simulink library "NCS_Library"  (R2019a)
settings: Solver=VariableStepAuto  StartTime=0.0  StopTime=10.0  RelTol=1e-3
values from neighbouring files (symbols this model uses):
  A = 10    [Parameter.m]
  band = 100000000    [Parameter.m]
  BER = 0    [Parameter.m]
  c = 5000000    [Parameter.m]
  c1 = 4.33    [Parameter.m]
  c2 = 3.16    [Parameter.m]
  CAN2EthernetDelay = 0.000    (= 0)    [Parameter.m]
  cR = 1.5*10^-3    (= 0.0015)    [Parameter.m]
  cw = (cwE * 2 + cwM * (nW_ges-2))/nW_ges    (= 0.1475)    [Parameter.m]
  cwE = 0.35    [Parameter.m]
  cwM = 0.08    [Parameter.m]
  Cycle_Controller = 0    [Parameter.m]
  CyclePLC = 24/1000    (= 0.024)    [Parameter.m]
  d = 800000    [Parameter.m]
  Dr = 0.92    [Parameter.m]
  Ethernet2CANDelay = 0.005    [Parameter.m]
  F_konst = 70892    [Parameter.m]
  FA = 100000    [Parameter.m]
  FB_WB_max = 10000    [Parameter.m]
  FBel_an = iG*nG*F_KZmax*nBan*R_mR/(Dr/2)    (= 28197.4297239)    [Parameter.m]
  FBel_frei = iG*nG*F_KZmax*nBfrei*R_mW/(Dr/2)    (= 29270.6882948)    [Parameter.m]
  Fmaxdyn = 300000    [Parameter.m]
  g = 9.81    [Parameter.m]
  i = 0    [Parameter.m]
  J = 1/2*mA*(Dr/2)^2    (= 158.7)    [Parameter.m]
  k1 = 0.095    [Parameter.m]
  k2 = 9.26/3.6    (= 2.57222222222)    [Parameter.m]
  k3 = 4.63/3.6    (= 1.28611111111)    [Parameter.m]
  mges = 58000    [Parameter.m]
  mu = [mu1 mu2]    [Parameter.m]
  muBel1 = 0.42    [Parameter.m]
  muBel2 = 0.36    [Parameter.m]
  n = 0.001    [Parameter.m]
  n_Mg = 4    [Parameter.m]
  n_WB = 4    [Parameter.m]
  nA = 4    [Parameter.m]
  nBan = 2    [Parameter.m]
  nBfrei = 3    [Parameter.m]
  nM = 4    [Parameter.m]
  nW_an = 4    [Parameter.m]
  P_max = 8200000    [Parameter.m]
  Q = 10    [Parameter.m]
  r_reib = 600    [Parameter.m]
  rho = 1.08    [Parameter.m]
  rhoL = 1.225    [Parameter.m]
  Size = 8    [Parameter.m]
  slip = [s1 s2]    [Parameter.m]
  tol = 0.05    [Parameter.m]
  v00 = 100/3.6    (= 27.7777777778)    [Parameter.m]
  v_grenz = 60/3.6    (= 16.6666666667)    [Parameter.m]
  v_opt = 75/3.6    (= 20.8333333333)    [Parameter.m]
  W_opt = 0.5    [Parameter.m]
  WB = 1    [Parameter.m]
  y_opt = sqrt(W_opt)/((1+sqrt(W_opt))^2+W_opt)    [Parameter.m]
undefined symbols (not defined in the file or in its folder): BUSCapacity, CableLength, controlGate, D_dyn, D_mg, EnableBurst, EnableToF, entity, Entity_out, Gate, Gate_4, Gate_5, Gate_ACK, Gate_copy, Gate_RX, getData, gettime, I_dyn, I_mg, m, magnitude, P_dyn, P_mg, ReadAttributes, readdata, ReadData, ReadSize, sigbuilder_block, Timeout, ToB, ToF, v0, v_d, v_soll
libraries: simulink x176, $bdroot x102
(part 8 of 12)

== system NCS_Library/Network/CAN/Logik/Slow_to_Fast/Logic Takt ==
  In : Inport
  Entity Takt : EntityGenerator  OutputPortMessageModes=m  TimeSource=Signal port  Period=7  AttributeName=entity  EntityTypeName=gate  EntityPriority=10  DataInitialValue=1
      settings: InputPortMap=u1
  Entity Terminator13 : EntityTerminator  InputPortMessageModes=m
  Gate : EntityGate  InputPortMessageModes=m,m  OutputPortMessageModes=m
  Offset [s] : Constant  Value=Offset
  Server : EntityServer  InputPortMessageModes=m  OutputPortMessageModes=m  Capacity=1  ServiceTimeValue=0  EntryAction=Gate(0);
  Server Offset : EntityServer  InputPortMessageModes=n,m  OutputPortMessageModes=m  Capacity=inf  ServiceTimeSource=Signal port  ServiceTimeValue=5
      settings: InputPortMap=u0,u2
  Server Takt : EntityServer  InputPortMessageModes=m  OutputPortMessageModes=m  Capacity=1  ServiceTimeValue=0.001  ServiceTimeAttributeName=CommDelay  EntryAction=Gate(Copy_on);  ExitAction=Gate(0);  SortingAttributeName=ID
  Simulink Function3 : Subsystem  TreatAsAtomicUnit=on
  Takt_fast [s] : Constant  Value=Takt_fast
  Out : Outport
  wires:
  Server/1 -> Out/1
  Gate/1 -> Server/1
  In/1 -> Gate/2
  Simulink Function3/1(ctrl) -> Gate/1
  Entity Takt/1 -> Server Offset/2
  Server Offset/1 -> Server Takt/1
  Server Takt/1 -> Entity Terminator13/1
  Takt_fast [s]/1 -> Entity Takt/1
  Offset [s]/1 -> Server Offset/1

== system NCS_Library/Network/CAN/Logik/Slow_to_Fast/Measurement ==
  measure : Inport
  Buffer_Measure : EntityQueue  InputPortMessageModes=m  OutputPortMessageModes=n,m  Capacity=1000  QueueType=LIFO  NumberEntitiesInBlock=on
      settings: OutputPortMap=o1,o5
  Detect Change : simulink/Logic and Bit Operations/Detect Change  vinit=0  OutDataTypeStr=boolean
  Digital Clock2 : DigitalClock  SampleTime=0.01
  Enabled Subsystem : Subsystem  TreatAsAtomicUnit=on
  Entity Replicator5 : EntityReplicator  InputPortMessageModes=m  OutputPortMessageModes=m,m
  Entity Terminator8 : EntityTerminator  InputPortMessageModes=m  EntryAction=getData(entity.Time)  NumberEntitiesArrived=on
      settings: OutputPortMap=o0
  Fast Takt : Subsystem
  Scope{,1,3,6} (4 alike) : Scope
  Simulink Function6 : Subsystem  TreatAsAtomicUnit=on
  Out : Outport
  wires:
  Digital Clock2/1 -> Enabled Subsystem/1(time_arrived)
  Simulink Function6/1(time) -> Enabled Subsystem/2(time), Scope3/1
  Detect Change/1 -> Enabled Subsystem/Enable
  Buffer_Measure/2 -> Fast Takt/1(In)
  Fast Takt/1(Out) -> Entity Replicator5/1
  Entity Terminator8/1 -> Detect Change/1, Scope6/1
  measure/1 -> Buffer_Measure/1
  Buffer_Measure/1 -> Scope1/1
  Enabled Subsystem/1(delay) -> Scope/1
  Entity Replicator5/2 -> Entity Terminator8/1
  Entity Replicator5/1 -> Out/1

== system NCS_Library/Network/CAN/Logik/Slow_to_Fast/Simulink Function1 ==
  Entity_out : TriggerPort  TriggerType=function-call  IsSimulinkFunction=on  FunctionName=Entity_out  FunctionVisibility=scoped  VariantControl=Variant
  Message Send : MessageSend  OutputPortMessageModes=m
      settings: InputPortMap=u1
  u : ArgIn  DisableCoverage=on  ArgumentName=u
  ctrl : Outport
  wires:
  u/1 -> Message Send/1
  Message Send/1 -> ctrl/1

== system NCS_Library/Network/CAN/Logik/Slow_to_Fast/Simulink Function3 ==
  Entity_in : TriggerPort  TriggerType=function-call  IsSimulinkFunction=on  FunctionName=Entity_in  FunctionVisibility=scoped  VariantControl=Variant
  Message Send : MessageSend  OutputPortMessageModes=m
      settings: InputPortMap=u1
  u : ArgIn  DisableCoverage=on  ArgumentName=u
  ctrl : Outport
  wires:
  Message Send/1 -> ctrl/1
  u/1 -> Message Send/1

== system NCS_Library/Network/ETB/Burst Device/Protocl Stack/TRDP PD ==
  note: Transmit
  note: Receive
  InFromSDTv2 : Inport
  Paramter : Inport  Port=2
  InFromUDP : Inport  Port=3
  Bus Selector : BusSelector  OutputSignals=T_Tx,SDTv2,msgType,Destination
  Bus Selector1 : BusSelector  OutputSignals=Address,Port,ReplyAddress
  Compare To Zero : simulink/Logic and Bit Operations/Compare To Zero  relop=>  OutDataTypeStr=boolean
  Constant : Constant  Value=0.0
  Constant2 : Constant
  Data Type Conversion : DataTypeConversion  OutDataTypeStr=uint8
  Detect Change : simulink/Logic and Bit Operations/Detect Change  vinit=0  OutDataTypeStr=boolean
  Display4 : Display
  Enabled Subsystem1 : Subsystem  TreatAsAtomicUnit=on
  Entity Server : EntityServer  InputPortMessageModes=n,m  OutputPortMessageModes=n,m  Capacity=1  ServiceTimeSource=Signal port  EntryAction=ReadData( entity.msgType, entity.ReplyAddress, entity.Source);  NumberEntitiesDeparted=on
      settings: InputPortMap=u0,u2  OutputPortMap=o0,o9
  Entity Server1 : EntityServer  InputPortMessageModes=m  OutputPortMessageModes=n,m  Capacity=1  ServiceTimeValue=0  EntryAction=[entity.SEQ, entity.msgType, entity.Destination, entity.Source, entity.CheckBit, entity.Data, entity.Port, entity.ReplyAddress] = SetAttributes(entity.SSC, entity.Data);  NumberEntitiesDeparted=on
      settings: OutputPortMap=o0,o9
  Message Send : MessageSend  OutputPortMessageModes=m  ShowEnablePort=on
      settings: InputPortMap=e0,u1
  Simulink Function : Subsystem  TreatAsAtomicUnit=on
  Simulink Function1 : Subsystem  TreatAsAtomicUnit=on
  Terminator{,1..3} (4 alike) : Terminator
  OutToSDTv2 : Outport
  TRM : Outport  Port=2
  #Transmit : Outport  Port=3
  msgType_transmit : Outport  Port=4
  #Receive : Outport  Port=5
  msgType_receive : Outport  Port=6
  OutToUDP : Outport  Port=7
  wires:
  Constant2/1 -> Message Send/2
  Message Send/1 -> TRM/1
  Bus Selector1/3 -> Simulink Function/5(ReplyAddress)  "<ReplyAddress>"
  Bus Selector1/2 -> Simulink Function/4(UDP)  "<Port>"
  Bus Selector1/1 -> Simulink Function/3(Source)  "<Address>"
  Bus Selector/3 -> Data Type Conversion/1  "<msgType>"
  Entity Server1/1 -> #Transmit/1
  Entity Server/1 -> Detect Change/1, #Receive/1
  Detect Change/1 -> Enabled Subsystem1/Enable
  Simulink Function1/2(ReplyAddress) -> Enabled Subsystem1/2(ReplyAddress)
  Simulink Function1/1(msgType) -> Enabled Subsystem1/1(msgType), msgType_receive/1
  InFromSDTv2/1 -> Entity Server1/1
  Entity Server1/2 -> OutToUDP/1
  Paramter/1 -> Bus Selector/1, Bus Selector1/1
  Constant/1 -> Entity Server/1
  Entity Server/2 -> OutToSDTv2/1
  Compare To Zero/1 -> Display4/1, Message Send/1
  Bus Selector/4 -> Simulink Function/2(Destination)  "<Destination>"
  InFromUDP/1 -> Entity Server/2
  Enabled Subsystem1/1(msgTypeReply) -> Terminator/1
  Enabled Subsystem1/2(DestinationReply) -> Terminator1/1
  Bus Selector/1 -> Terminator2/1  "<T_Tx>"
  Bus Selector/2 -> Terminator3/1  "<SDTv2>"
  Data Type Conversion/1 -> Compare To Zero/1, msgType_transmit/1, Simulink Function/1(msgType)

== system NCS_Library/Network/ETB/Controller Interface/Subsystem/Transport Layers ==
  InFromApplication4 : Inport
  InFromApplication3 : Inport  Port=2
  InFromApplication2 : Inport  Port=3
  InFromApplication1 : Inport  Port=4
  Parameter : Inport  Port=5
  RxFromBus : Inport  Port=6
  CycleRx : EntityServer  InputPortMessageModes=m  OutputPortMessageModes=m  Capacity=100  ServiceTimeValue=CycleRx
  CycleTx : EntityServer  InputPortMessageModes=m  OutputPortMessageModes=m  Capacity=100  ServiceTimeValue=CycleTx
  Entity Generator1 : EntityGenerator  InputPortMessageModes=m  OutputPortMessageModes=m  GenerationMethod=Event-based  TimeSource=Signal port  GenerateEntityAtSimulationStart=off  EntityType=Bus object  EntityTypeName=Ethernet_Entity
      settings: InputPortMap=u0
  Entity Replicator : EntityReplicator  InputPortMessageModes=m  OutputPortMessageModes=m,m,m,m  NumberReplicas=3
      settings: OutputPortMap=o0,o1,o2,o3
  Entity Terminator{3..6} (4 alike) : EntityTerminator  InputPortMessageModes=m
  Ground1 : Ground
  IP : $bdroot/Network/ETB/OSI Layers/IP  SystemSampleTime=-1
  MAC Controller : $bdroot/Network/ETB/OSI Layers/MAC Controller  SystemSampleTime=-1
  Parameter1 : InportShadow  Port=5
  Terminator : Terminator
  Terminator1 : Terminator
  UDP Multi-Port : $bdroot/Network/ETB/OSI Layers/UDP Multi-Port  SystemSampleTime=-1
  OutToApplication4 : Outport
  OutToApplication3 : Outport  Port=2
  OutToApplication2 : Outport  Port=3
  OutToApplication1 : Outport  Port=4
  Delay : Outport  Port=5
  #damaged : Outport  Port=6
  TxToBus : Outport  Port=7
  wires:
  Parameter/1 -> MAC Controller/2
  RxFromBus/1 -> MAC Controller/3
  MAC Controller/4 -> TxToBus/1
  Parameter1/1 -> IP/2
  MAC Controller/2 -> Terminator/1  "#collision"
  MAC Controller/3 -> Terminator1/1  "Retry"
  UDP Multi-Port/9 -> IP/1
  IP/1 -> UDP Multi-Port/9
  UDP Multi-Port/1 -> OutToApplication1/1
  Entity Generator1/1 -> Entity Replicator/1
  UDP Multi-Port/5 -> Entity Terminator3/1
  UDP Multi-Port/6 -> Entity Terminator4/1
  UDP Multi-Port/7 -> Entity Terminator5/1
  UDP Multi-Port/8 -> Entity Terminator6/1
  Ground1/1 -> Entity Generator1/1
  InFromApplication1/1 -> UDP Multi-Port/1
  InFromApplication2/1 -> UDP Multi-Port/2
  InFromApplication3/1 -> UDP Multi-Port/3
  InFromApplication4/1 -> UDP Multi-Port/4
  Entity Replicator/1 -> UDP Multi-Port/5
  Entity Replicator/2 -> UDP Multi-Port/6
  Entity Replicator/3 -> UDP Multi-Port/7
  Entity Replicator/4 -> UDP Multi-Port/8
  UDP Multi-Port/3 -> OutToApplication3/1
  UDP Multi-Port/4 -> OutToApplication4/1
  UDP Multi-Port/2 -> OutToApplication2/1
  IP/4 -> CycleTx/1
  CycleTx/1 -> MAC Controller/1
  CycleRx/1 -> IP/3
  MAC Controller/1 -> CycleRx/1
  IP/3 -> Delay/1  "delay"
  IP/2 -> #damaged/1

== system NCS_Library/Network/ETB/ED/Protocol Stack/Simulink Function ==
  f : TriggerPort  TriggerType=function-call  IsSimulinkFunction=on  FunctionName=ReadSize  FunctionVisibility=scoped  VariantControl=(inherit)
  u : ArgIn  DisableCoverage=on  ArgumentName=Size
  Out1 : Outport
  wires:
  u/1 -> Out1/1

== system NCS_Library/Network/ETB/ED/Protocol Stack/Subsystem ==
  Signal : Inport
  Data : Inport  Port=2
  In3 : Inport  Port=3
  Phase : Inport  Port=4
  In5 : Inport  Port=5
  In6 : Inport  Port=6
  In7 : Inport  Port=7
  In8 : Inport  Port=8
  In9 : Inport  Port=9
  delay : Inport  Port=10
  #collision : Inport  Port=11
  Retry : Inport  Port=12
  SDTv2 : Inport  Port=13
  Bus Creator1 : BusCreator  Commented=on  Inputs=13
  Data Type Conversion{,1..6} (7 alike) : DataTypeConversion  OutDataTypeStr=double
  Detect Change : simulink/Logic and Bit Operations/Detect Change  vinit=0  OutDataTypeStr=boolean
  Out1 : Outport
  wires:
  SDTv2/1 -> Bus Creator1/13  "SDTv2"
  Data Type Conversion/1 -> Bus Creator1/6  "msgType_transmit"
  Signal/1 -> Bus Creator1/1
  Data Type Conversion5/1 -> Bus Creator1/9  "#damaged"
  Data Type Conversion6/1 -> Bus Creator1/7  "#Receive"
  Data Type Conversion1/1 -> Bus Creator1/5  "#Transmit"
  In7/1 -> Data Type Conversion6/1
  Data Type Conversion3/1 -> Bus Creator1/3  "SSC"
  Data Type Conversion2/1 -> Bus Creator1/8  "msgType_receive"
  Data Type Conversion4/1 -> Bus Creator1/12  "Retry"
  Detect Change/1 -> Data Type Conversion4/1
  In6/1 -> Data Type Conversion/1
  Data/1 -> Bus Creator1/2
  In9/1 -> Data Type Conversion5/1
  In3/1 -> Data Type Conversion3/1
  #collision/1 -> Bus Creator1/11
  In8/1 -> Data Type Conversion2/1
  In5/1 -> Data Type Conversion1/1
  delay/1 -> Out1/1, Bus Creator1/10
  Retry/1 -> Detect Change/1
  Phase/1 -> Bus Creator1/4

== system NCS_Library/Network/ETB/ED/User Interface/Subsystem2 ==
  In1 : Inport
  MATLAB Function : MATLAB Function  TreatAsAtomicUnit=on
  Out1 : Outport
  wires:
  MATLAB Function/1(y) -> Out1/1
  In1/1 -> MATLAB Function/1(u)

== system NCS_Library/Network/ETB/OSI Layers/Application/Edit Paramter ==
  UDP_Port : Inport
  Parameter : Inport  Port=2
  Bus Creator : BusCreator  Inputs=8
  Bus Selector : BusSelector  OutputSignals=Address,Destination,Subscribe,ReplyAddress,Port,T_Tx,msgType,SDTv2
  Display : Display
  MATLAB Function : MATLAB Function  TreatAsAtomicUnit=on
  MATLAB Function1 : MATLAB Function  TreatAsAtomicUnit=on
  MATLAB Function2 : MATLAB Function  TreatAsAtomicUnit=on
  MATLAB Function3 : MATLAB Function  TreatAsAtomicUnit=on
  Terminator : Terminator
  UDP_Port{1..4} (4 alike) : InportShadow
  Parameter_edited : Outport
  wires:
  Parameter/1 -> Bus Selector/1
  Bus Creator/1 -> Parameter_edited/1
  Bus Selector/6 -> MATLAB Function1/2(In)  "<T_Tx>"
  Bus Selector/3 -> Bus Creator/3  "<Subscribe>"
  Bus Selector/1 -> Bus Creator/1  "<Address>"
  Bus Selector/8 -> MATLAB Function3/2(In)  "<SDTv2>"
  Bus Selector/2 -> MATLAB Function/2(U)  "<Destination>"
  MATLAB Function/1(y) -> Display/1, Bus Creator/2  "Destination"
  UDP_Port/1 -> MATLAB Function/1(UDP)  "Port"
  UDP_Port1/1 -> Bus Creator/5  "Port"
  Bus Selector/5 -> Terminator/1  "<Port>"
  MATLAB Function1/1(Value) -> Bus Creator/6  "T_Tx"
  UDP_Port2/1 -> MATLAB Function1/1(Port)  "Port"
  MATLAB Function2/1(Value) -> Bus Creator/7  "msgType"
  Bus Selector/7 -> MATLAB Function2/2(In)  "<msgType>"
  UDP_Port3/1 -> MATLAB Function2/1(Port)  "Port"
  MATLAB Function3/1(Value) -> Bus Creator/8  "SDTv2"
  UDP_Port4/1 -> MATLAB Function3/1(Port)  "Port"
  Bus Selector/4 -> Bus Creator/4  "<ReplyAddress>"

== system NCS_Library/Network/ETB/OSI Layers/Application/Receive Sensor Data ==
  Parameter : Inport
  InFromUDP : Inport  Port=2
  Bus Selector : BusSelector  OutputSignals=SDTv2,T_Tx,msgType
  Entity Terminator : EntityTerminator  InputPortMessageModes=m
  Ground : Ground
  Ground2 : Ground
  SDTv2 : $bdroot/Network/ETB/OSI Layers/SDTv2  SystemSampleTime=-1
  TRDP PD : $bdroot/Network/ETB/OSI Layers/TRDP PD  SystemSampleTime=-1
  Terminator{,1..5} (6 alike) : Terminator
  OutToController : Outport
  wires:
  SDTv2/4 -> TRDP PD/1
  TRDP PD/2 -> SDTv2/6
  Bus Selector/3 -> SDTv2/4  "<msgType>"
  TRDP PD/1 -> SDTv2/5
  Bus Selector/1 -> SDTv2/2  "<SDTv2>"
  Bus Selector/2 -> SDTv2/3  "<T_Tx>"
  SDTv2/1 -> OutToController/1  "Y_M"
  InFromUDP/1 -> TRDP PD/4
  TRDP PD/7 -> Entity Terminator/1
  SDTv2/2 -> Terminator/1
  SDTv2/3 -> Terminator1/1
  Ground/1 -> SDTv2/1
  TRDP PD/6 -> Terminator5/1
  TRDP PD/5 -> Terminator2/1
  TRDP PD/4 -> Terminator3/1
  TRDP PD/3 -> Terminator4/1
  Parameter/1 -> TRDP PD/3, Bus Selector/1
  Ground2/1 -> TRDP PD/2

== system NCS_Library/Network/ETB/OSI Layers/Application/Simulink Function ==
  Sort : TriggerPort  TriggerType=function-call  IsSimulinkFunction=on  FunctionName=Sort  FunctionVisibility=scoped  VariantControl=(inherit)
  Add : Sum
  Compare To Constant : simulink/Logic and Bit Operations/Compare To Constant  relop===  const=11  OutDataTypeStr=uint8
  Constant : Constant  OutDataTypeStr=uint8
  u : ArgIn  DisableCoverage=on  OutDataTypeStr=uint8  ArgumentName=msgType
  y : ArgOut  DisableCoverage=on  OutDataTypeStr=uint8  ArgumentName=Route
  wires:
  u/1 -> Compare To Constant/1
  Compare To Constant/1 -> Add/1  "Request"
  Add/1 -> y/1
  Constant/1 -> Add/2

== system NCS_Library/Network/ETB/OSI Layers/Application/Transmit Actuator Data ==
  InFromController : Inport
  InFromUDP : Inport  Port=2
  Parameter : Inport  Port=3
  Bus Selector : BusSelector  OutputSignals=SDTv2,T_Tx,msgType
  Parameter1 : InportShadow  Port=3
  SDTv2 : $bdroot/Network/ETB/OSI Layers/SDTv2  SystemSampleTime=-1
  TRDP PD : $bdroot/Network/ETB/OSI Layers/TRDP PD  SystemSampleTime=-1
  Terminator{,1..6} (7 alike) : Terminator
  OutToUDP : Outport
  wires:
  Parameter/1 -> Bus Selector/1
  Bus Selector/2 -> SDTv2/3  "<T_Tx>"
  Bus Selector/1 -> SDTv2/2  "<SDTv2>"
  Bus Selector/3 -> SDTv2/4  "<msgType>"
  InFromController/1 -> TRDP PD/2, SDTv2/1
  TRDP PD/1 -> SDTv2/5
  TRDP PD/2 -> SDTv2/6
  SDTv2/4 -> TRDP PD/1
  TRDP PD/7 -> OutToUDP/1
  InFromUDP/1 -> TRDP PD/4
  TRDP PD/3 -> Terminator/1
  TRDP PD/4 -> Terminator1/1
  TRDP PD/5 -> Terminator2/1
  TRDP PD/6 -> Terminator3/1
  SDTv2/3 -> Terminator4/1  "Phase"
  SDTv2/2 -> Terminator5/1
  SDTv2/1 -> Terminator6/1  "Data"
  Parameter1/1 -> TRDP PD/3

== system NCS_Library/Network/ETB/OSI Layers/IP/Simulink Function ==
  time : Inport
  SetAttributes : TriggerPort  TriggerType=function-call  IsSimulinkFunction=on  FunctionName=SetAttributes  FunctionVisibility=scoped  VariantControl=(inherit)
  Display : Display
  Display4 : Display
  MATLAB Function : MATLAB Function  TreatAsAtomicUnit=on
  Destination : ArgIn  OutDataTypeStr=uint16  PortDimensions=[ 1 4]  ArgumentName=Destination
  Source : ArgIn  Port=2  OutDataTypeStr=uint16  PortDimensions=[1 4 ]  ArgumentName=Source
  Timestamp : ArgOut  DisableCoverage=on  ArgumentName=Timestamp
  MACDestination : ArgOut  DisableCoverage=on  Port=2  OutDataTypeStr=uint16  ArgumentName=MACDestination
  MACSource : ArgOut  DisableCoverage=on  Port=3  OutDataTypeStr=uint16  ArgumentName=MACSource
  wires:
  time/1 -> Timestamp/1
  Destination/1 -> MATLAB Function/2(Destination)
  Source/1 -> MATLAB Function/1(Source)
  MATLAB Function/2(MACDestination) -> Display/1, MACDestination/1
  MATLAB Function/1(MACSource) -> Display4/1, MACSource/1

== system NCS_Library/Network/ETB/OSI Layers/IP/Simulink Function1 ==
  Address : Inport
  SN : Inport  Port=2
  getAttributes : TriggerPort  TriggerType=function-call  IsSimulinkFunction=on  FunctionName=getAttributes  FunctionVisibility=scoped  VariantControl=(inherit)
  Display{1..4} (4 alike) : Display
  MATLAB Function : MATLAB Function  TreatAsAtomicUnit=on
  Destination2 : ArgIn  ArgumentName=Timestamp
  Source1 : ArgIn  Port=2  OutDataTypeStr=uint16  PortDimensions=[1 4 ]  ArgumentName=Source
  Destination1 : ArgIn  Port=3  OutDataTypeStr=uint16  PortDimensions=[ 1 4]  ArgumentName=Destination
  Route : ArgOut  DisableCoverage=on  OutDataTypeStr=uint8  ArgumentName=Route
  Timestamp : Outport
  Source : Outport  Port=2
  Destination : Outport  Port=3
  wires:
  Destination2/1 -> Timestamp/1
  MATLAB Function/1(Route) -> Route/1
  Address/1 -> Display2/1, MATLAB Function/1(Address)
  SN/1 -> Display4/1, MATLAB Function/4(SN)
  Source1/1 -> Source/1, Display1/1, MATLAB Function/2(Source)
  Destination1/1 -> Destination/1, Display3/1, MATLAB Function/3(Destination)

== system NCS_Library/Network/ETB/OSI Layers/IP/Subsystem ==
  delay : Inport
  Source : Inport  Port=2
  Destination : Inport  Port=3
  Enable : EnablePort
  Data Type Conversion : DataTypeConversion  OutDataTypeStr=double
  Data Type Conversion1 : DataTypeConversion  OutDataTypeStr=double
  Mux : Mux  Inputs=3
  DELAY : Outport  OutputWhenDisabled=reset  InitialOutput=0
  wires:
  delay/1 -> Mux/1
  Source/1 -> Data Type Conversion/1
  Destination/1 -> Data Type Conversion1/1
  Mux/1 -> DELAY/1
  Data Type Conversion/1 -> Mux/2
  Data Type Conversion1/1 -> Mux/3

== system NCS_Library/Network/ETB/OSI Layers/MAC Controller/BckOffCntrl ==
  Address : Inport
  bckoffctrl : TriggerPort  TriggerType=function-call  IsSimulinkFunction=on  FunctionName=bckoffctrl  FunctionVisibility=scoped  VariantControl=Variant
  Display{,1..5} (6 alike) : Display
  MATLAB Function : MATLAB Function  TreatAsAtomicUnit=on
  Memory1 : Memory  InheritSampleTime=on
  NumC : ArgIn  OutDataTypeStr=uint8  ArgumentName=NumC
  Coll : ArgIn  Port=2  OutDataTypeStr=uint8  ArgumentName=Coll
  MACSource : ArgIn  Port=3  OutDataTypeStr=uint16  ArgumentName=MACSource
  MACDestination : ArgIn  Port=4  OutDataTypeStr=uint16  ArgumentName=MACDestination
  SEQ : ArgIn  Port=5  OutDataTypeStr=uint32  ArgumentName=SEQ
  SEQ1 : ArgIn  Port=6  ArgumentName=ServiceTime
  Route : ArgOut  DisableCoverage=on  OutDataTypeStr=uint8  ArgumentName=Route
  NumCollision : ArgOut  DisableCoverage=on  Port=2  OutDataTypeStr=uint8  ArgumentName=NumCollision
  BOTime : ArgOut  DisableCoverage=on  Port=3  ArgumentName=BOTime
  #collision : Outport
  wires:
  Memory1/1 -> MATLAB Function/1("n_collision ")
  MATLAB Function/2(route) -> Display4/1, Route/1
  MATLAB Function/4(numColl) -> NumCollision/1
  NumC/1 -> MATLAB Function/2("numColl ")
  Coll/1 -> Display5/1, MATLAB Function/4(collision)
  MACSource/1 -> Display1/1, MATLAB Function/5(MACSource)
  MACDestination/1 -> Display3/1, MATLAB Function/6(MACDestination)
  SEQ/1 -> MATLAB Function/8(SEQ)
  MATLAB Function/3(bckoffTime) -> Display2/1, BOTime/1
  MATLAB Function/1(n_collision) -> #collision/1, Memory1/1
  Address/1 -> Display/1, MATLAB Function/3(Address)
  SEQ1/1 -> MATLAB Function/7(SlotTime)

== system NCS_Library/Network/ETB/OSI Layers/MAC Controller/CSMA//CD ==
  note: This subsystem aims to determine whether a packet is the only packet on the communication channel for the entire duration of transmission.
      |
      | The l_status input signal is the number of packets in a server in the parent system (Ethernet MAC Controller). The S-R Flip-Flop block responds
      | to these events:
      |
      |     -- If l_status increases from 0 to 1, then
      |        -- R has a rising edge.
      |        -- The S-R Flip-Flop gets reset
      |        -- The S-R Flip-Floo output signal becomes 0.
      |
      |     -- If l_status increases from 1 to 2, then
      |         -- S has a rising edge.
      |         -- The S-R Flip-Flop gets set
      |         -- The S-R Flip-Flop block's st output signal becomes 1.
      |
      | By the time the packet departs from the server in the parent system, the Signal Latch block's st signal is 0 if and only if that packet has been the
      | only packet in the server block for the entire duration of service. This outcome represents a success for that packet. Other outcomes represent
      | collisions between that packet and one or more other packets.
  l_status : Inport
  Discrete Event Subsystem (Carrier Sensing)1 : Subsystem  TreatAsAtomicUnit=on
  Scope : Scope
  Scope1 : Scope
  l_ready : Outport
  wires:
  l_status/1 -> Discrete Event Subsystem (Carrier Sensing)1/1(l_status), Scope/1
  Discrete Event Subsystem (Carrier Sensing)1/1(l_ready) -> l_ready/1, Scope1/1

== system NCS_Library/Network/ETB/OSI Layers/MAC Controller/CSMA//CD Entry ==
  l_status : Inport
  Entry : TriggerPort  TriggerType=function-call  IsSimulinkFunction=on  FunctionName=Entry  FunctionVisibility=scoped  VariantControl=Variant
  Display : Display
  MATLAB Function : MATLAB Function  TreatAsAtomicUnit=on
  Coll : ArgIn  OutDataTypeStr=uint8  ArgumentName=Coll
  pck_ok : ArgOut  DisableCoverage=on  OutDataTypeStr=uint8  ArgumentName=Collision
  wires:
  l_status/1 -> MATLAB Function/1(n)
  Coll/1 -> MATLAB Function/2("collision ")
  MATLAB Function/1(collision) -> Display/1, pck_ok/1

== system NCS_Library/Network/ETB/OSI Layers/MAC Controller/CSMA//CD Exit ==
  l_status : Inport
  Exit : TriggerPort  TriggerType=function-call  IsSimulinkFunction=on  FunctionName=Exit  FunctionVisibility=scoped  VariantControl=Variant
  Display : Display
  MATLAB Function : MATLAB Function  TreatAsAtomicUnit=on
  Coll : ArgIn  OutDataTypeStr=uint8  ArgumentName=Coll
  Collision : ArgOut  DisableCoverage=on  OutDataTypeStr=uint8  ArgumentName=Collision
  wires:
  Coll/1 -> MATLAB Function/2("collision ")
  l_status/1 -> MATLAB Function/1(n)
  MATLAB Function/1(collision) -> Display/1, Collision/1

== system NCS_Library/Network/ETB/OSI Layers/MAC Controller/Simulink Function1 ==
  f : TriggerPort  TriggerType=function-call  IsSimulinkFunction=on  FunctionName=SetServiceTime  FunctionVisibility=scoped  VariantControl=(inherit)
  Display : Display
  Display1 : Display
  Gain : Gain  Gain=1/band
  MACSource : ArgIn  ArgumentName=Size
  y : ArgOut  DisableCoverage=on  ArgumentName=ServiceTime
  wires:
  MACSource/1 -> Display1/1, Gain/1
  Gain/1 -> Display/1, y/1

== system NCS_Library/Network/ETB/OSI Layers/MAC Controller/Transmission Buffer Control ==
  #success : Inport
  #failure : Inport  Port=2
  Constant : Constant
  Detect Change : simulink/Logic and Bit Operations/Detect Change  vinit=0  OutDataTypeStr=boolean
  Detect Change1 : simulink/Logic and Bit Operations/Detect Change  vinit=0  OutDataTypeStr=boolean
  Display{,1..4} (5 alike) : Display
  Entity Server : EntityServer  InputPortMessageModes=m  OutputPortMessageModes=n,m  Capacity=1  ServiceTimeValue=0  NumberEntitiesDeparted=on
      settings: OutputPortMap=o0,o9
  Logical Operator : Logic  Operator=OR  AllPortsSameDT=off  OutDataTypeStr=boolean
  Message Send : MessageSend  OutputPortMessageModes=m  ShowEnablePort=on
      settings: InputPortMap=e0,u1
  state : Outport
  wires:
  Entity Server/2 -> state/1
  Entity Server/1 -> Display4/1
  Message Send/1 -> Entity Server/1
  Logical Operator/1 -> Message Send/1
  #failure/1 -> Detect Change1/1, Display3/1
  Constant/1 -> Message Send/2
  #success/1 -> Detect Change/1, Display/1
  Detect Change/1 -> Display1/1, Logical Operator/1
  Detect Change1/1 -> Display2/1, Logical Operator/2

== system NCS_Library/Network/ETB/OSI Layers/SDTv2/Get Phase ==
  LSC : Inport
  Init : Inport  Port=2
  Contraction : Inport  Port=3
  MATLAB Function : MATLAB Function  TreatAsAtomicUnit=on
  Memory : Memory  InheritSampleTime=on
  Phase : Outport
  wires:
  Contraction/1 -> MATLAB Function/3(Contraction)
  LSC/1 -> MATLAB Function/2(LSC)
  MATLAB Function/1(Phase) -> Memory/1, Phase/1
  Init/1 -> MATLAB Function/4(Init)
  Memory/1 -> MATLAB Function/1(Phase_previous)

== system NCS_Library/Network/ETB/OSI Layers/SDTv2/Safety Measures ==
  Timestamp : Inport
  SCC : Inport  Port=2
  T_rx_safe : Inport  Port=3
  Compare To Zero : simulink/Logic and Bit Operations/Compare To Zero  relop=>  OutDataTypeStr=boolean
  Display : Display
  Latency Monitoring : Subsystem
  Sink-Time Supervision : Subsystem
  Subsystem : Subsystem
  LSC : Outport
  Init : Outport  Port=2
  Contraction Phase : Outport  Port=3
  wires:
  Sink-Time Supervision/1(LSC) -> LSC/1
  Latency Monitoring/1(Contration Phase) -> Contraction Phase/1
  T_rx_safe/1 -> Display/1, Sink-Time Supervision/1(T_rx_safe), Latency Monitoring/2(T_rx_safe)
  SCC/1 -> Sink-Time Supervision/2(SSC), Subsystem/1(In1), Compare To Zero/1
  Compare To Zero/1 -> Init/1
  Timestamp/1 -> Latency Monitoring/1(Timestamp)
  Subsystem/1(Out1) -> Latency Monitoring/Enable

== system NCS_Library/Network/ETB/OSI Layers/SDTv2/Simulink Function ==
  InData : Inport
  T_tx : Inport  Port=2
  In1 : Inport  Port=3
  SetAttributes : TriggerPort  TriggerType=function-call  IsSimulinkFunction=on  FunctionName=SetAttributes  FunctionVisibility=scoped  VariantControl=(inherit)
  Add : Sum
  Constant : Constant  OutDataTypeStr=uint32
  Constant1 : Constant  Value=Size  OutDataTypeStr=double
  Data Type Conversion : DataTypeConversion  OutDataTypeStr=uint32
  Display : Display
  Display1 : Display
  Gain : Gain  Gain=8
  SSC : ArgOut  DisableCoverage=on  OutDataTypeStr=uint32  ArgumentName=SSC
  Data : ArgOut  DisableCoverage=on  Port=2  PortDimensions=[3 20]  ArgumentName=Data
  Size1 : ArgOut  DisableCoverage=on  Port=3  ArgumentName=T_Tx
  Size : ArgOut  DisableCoverage=on  Port=4  ArgumentName=Size
  wires:
  InData/1 -> Display/1, Data/1
  In1/1 -> Data Type Conversion/1
  Add/1 -> SSC/1
  Constant/1 -> Add/2
  Data Type Conversion/1 -> Add/1
  Constant1/1 -> Gain/1
  T_tx/1 -> Size1/1
  Gain/1 -> Display1/1, Size/1

== system NCS_Library/Network/ETB/OSI Layers/SDTv2/Simulink Function1 ==
  SSC_last : Inport  OutDataTypeStr=uint32
  SDTv2 : Inport  Port=2
  Check : TriggerPort  TriggerType=function-call  IsSimulinkFunction=on  FunctionName=Check  FunctionVisibility=scoped  VariantControl=(inherit)
  Constant : Constant  OutDataTypeStr=uint8
  MATLAB Function : MATLAB Function  TreatAsAtomicUnit=on
  Switch1 : Switch  Criteria=u2 > Threshold
  u : ArgIn  DisableCoverage=on  OutDataTypeStr=uint32  ArgumentName=SSC
  u1 : ArgIn  DisableCoverage=on  Port=2  ArgumentName=T_tx
  y : ArgOut  DisableCoverage=on  OutDataTypeStr=uint8  ArgumentName=Route
  SSC : Outport  OutDataTypeStr=uint32  InitialOutput=0
  T_tx : Outport  Port=2  InitialOutput=0
  wires:
  u/1 -> MATLAB Function/2(SSC)
  SSC_last/1 -> MATLAB Function/1(SSC_last)
  MATLAB Function/1(SSC_received) -> SSC/1
  SDTv2/1 -> Switch1/2
  Constant/1 -> Switch1/3
  u1/1 -> T_tx/1
  Switch1/1 -> y/1
  MATLAB Function/2(Route) -> Switch1/1

== system NCS_Library/Network/ETB/OSI Layers/SDTv2/Simulink Function2 ==
  ReadAttributes : TriggerPort  TriggerType=function-call  IsSimulinkFunction=on  FunctionName=ReadAttributes  FunctionVisibility=scoped  VariantControl=(inherit)
  Display : Display
  SSC : ArgIn  DisableCoverage=on  OutDataTypeStr=uint32  ArgumentName=SSC
  Data : ArgIn  DisableCoverage=on  Port=2  PortDimensions=[3 20]  ArgumentName=Data
  Data1 : ArgIn  DisableCoverage=on  Port=3  ArgumentName=Timestamp
  OutTime : Outport
  OutSSC : Outport  Port=2
  OutData : Outport  Port=3
  wires:
  SSC/1 -> OutSSC/1  "SSC"
  Data/1 -> Display/1, OutData/1  "Data"
  Data1/1 -> OutTime/1  "Timestamp"

== system NCS_Library/Network/ETB/OSI Layers/SDTv2/Subsystem ==
  T_Rx : Inport
  Add1 : Sum  Inputs=+--+
  Clock : Clock
  Compare To Zero1 : simulink/Logic and Bit Operations/Compare To Zero  relop=>=  OutDataTypeStr=uint8
  Constant : Constant  Value=1e-10
  Constant1 : Constant
  Display{,2..3,5..6} (5 alike) : Display
  IC : InitialCondition
  Memory : Memory  InheritSampleTime=on
  Message Send : MessageSend  OutputPortMessageModes=m  ShowEnablePort=on
      settings: InputPortMap=e0,u1
  Multiply : Product
  Save last release time : Subsystem
  T_Rx2 : InportShadow
  Out1 : Outport
  wires:
  Add1/1 -> Display2/1, Compare To Zero1/1
  Clock/1 -> Display/1, Add1/1
  Compare To Zero1/1 -> IC/1, Display5/1, Save last release time/Enable
  Constant/1 -> Add1/4  "Compensate numeric drift"
  T_Rx/1 -> Add1/3
  Save last release time/1(Out1) -> Memory/1
  T_Rx2/1 -> Multiply/1
  Multiply/1 -> Display3/1, Add1/2
  Memory/1 -> Display6/1, Multiply/2, Save last release time/1(Time)
  Message Send/1 -> Out1/1
  IC/1 -> Message Send/1
  Constant1/1 -> Message Send/2

== system NCS_Library/Network/ETB/OSI Layers/TRDP PD/Detect Event ==
  Data : Inport
  Constant : Constant
  DetectEvent : MATLAB Function  TreatAsAtomicUnit=on
  Display : Display
  Enabled Subsystem : Subsystem  TreatAsAtomicUnit=on
  Memory : Memory
  Event : Outport
  wires:
  Enabled Subsystem/1(Out1) -> Event/1
  Constant/1 -> Enabled Subsystem/1(In1)
  Data/1 -> DetectEvent/1(U)
  DetectEvent/1(Change) -> Enabled Subsystem/Enable, Display/1
  Memory/1 -> DetectEvent/2(Memory)
  DetectEvent/2(M) -> Memory/1

== system NCS_Library/Network/ETB/OSI Layers/TRDP PD/Enabled Subsystem1 ==
  msgType : Inport
  ReplyAddress : Inport  Port=2
  Enable : EnablePort
  MATLAB Function : MATLAB Function  TreatAsAtomicUnit=on
  msgTypeReply : Outport  OutputWhenDisabled=reset  InitialOutput=0
  DestinationReply : Outport  Port=2
  wires:
  msgType/1 -> MATLAB Function/1(msgType)
  ReplyAddress/1 -> DestinationReply/1
  MATLAB Function/1(msgTypeReply) -> msgTypeReply/1

== system NCS_Library/Network/ETB/OSI Layers/TRDP PD/Simulink Function ==
  msgType : Inport
  Destination : Inport  Port=2
  Source : Inport  Port=3
  UDP : Inport  Port=4
  ReplyAddress : Inport  Port=5
  f : TriggerPort  TriggerType=function-call  IsSimulinkFunction=on  FunctionName=SetAttributes  FunctionVisibility=scoped  VariantControl=(inherit)
  Constant : Constant  OutDataTypeStr=uint8
  Display : Display
  MATLAB Function : MATLAB Function  TreatAsAtomicUnit=on
  SSC : ArgIn  DisableCoverage=on  OutDataTypeStr=uint32  ArgumentName=SSC
  SSC1 : ArgIn  DisableCoverage=on  Port=2  PortDimensions=[ 3 20]  ArgumentName=Data
  y : ArgOut  DisableCoverage=on  OutDataTypeStr=uint32  ArgumentName=SEQ
  y1 : ArgOut  DisableCoverage=on  Port=2  OutDataTypeStr=uint8  ArgumentName=msgType
  y2 : ArgOut  DisableCoverage=on  Port=3  OutDataTypeStr=uint16  PortDimensions=[1 4]  ArgumentName=Destination
  y3 : ArgOut  DisableCoverage=on  Port=4  OutDataTypeStr=uint16  PortDimensions=[1 4]  ArgumentName=Source
  y5 : ArgOut  DisableCoverage=on  Port=5  OutDataTypeStr=uint8  ArgumentName=CheckBit
  y4 : ArgOut  DisableCoverage=on  Port=6  PortDimensions=[3 20]  ArgumentName=Data
  y6 : ArgOut  DisableCoverage=on  Port=7  OutDataTypeStr=uint16  ArgumentName=UDP
  y7 : ArgOut  DisableCoverage=on  Port=8  OutDataTypeStr=uint16  PortDimensions=[ 1 4 ]  ArgumentName=ReplyAddress
  wires:
  msgType/1 -> MATLAB Function/2(msgType), y1/1
  Destination/1 -> Display/1, y2/1
  Source/1 -> y3/1
  SSC/1 -> y/1
  Constant/1 -> y5/1
  SSC1/1 -> MATLAB Function/1(Data)
  MATLAB Function/1(Data_edited) -> y4/1
  UDP/1 -> y6/1
  ReplyAddress/1 -> y7/1

== system NCS_Library/Network/ETB/OSI Layers/TRDP PD/Simulink Function1 ==
  ReadData : TriggerPort  TriggerType=function-call  IsSimulinkFunction=on  FunctionName=ReadData  FunctionVisibility=scoped  VariantControl=(inherit)
  MATLAB Function : MATLAB Function  TreatAsAtomicUnit=on
  MATLAB Function2 : MATLAB Function  TreatAsAtomicUnit=on
  SourceAddress : ArgIn  DisableCoverage=on  OutDataTypeStr=uint8  ArgumentName=msgType
  SourceAddress1 : ArgIn  DisableCoverage=on  Port=2  OutDataTypeStr=uint16  PortDimensions=[1 4]  ArgumentName=Reply
  SourceAddress2 : ArgIn  DisableCoverage=on  Port=3  OutDataTypeStr=uint16  PortDimensions=[1 4]  ArgumentName=Source
  msgType : Outport  OutDataTypeStr=uint8  OutputWhenDisabled=reset  InitialOutput=0
  ReplyAddress : Outport  Port=2  OutDataTypeStr=uint16
  wires:
  SourceAddress1/1 -> MATLAB Function/1(Reply)
  SourceAddress2/1 -> MATLAB Function/2(Source)
  MATLAB Function/1(Address) -> MATLAB Function2/2(ReplyAddress)
  SourceAddress/1 -> msgType/1, MATLAB Function2/1(msgType)
  MATLAB Function2/1(DestinationPull) -> ReplyAddress/1

== system NCS_Library/Network/ETB/OSI Layers/TRDP PD/Subsystem ==
  T_signal : Inport
  SDTv2 : Inport  Port=2
  Add1 : Sum  Inputs=+--+
  Clock : Clock
  Compare To Zero1 : simulink/Logic and Bit Operations/Compare To Zero  relop=>=  OutDataTypeStr=uint8
  Constant : Constant  Value=1e-10
  Display{,2..3,5..6} (5 alike) : Display
  Gain : Gain  Gain=1/3
  IC : InitialCondition  Value=0
  Memory : Memory  InheritSampleTime=on
  Multiply : Product
  Save last release time : Subsystem
  Switch : Switch  Criteria=u2 > Threshold
  Out1 : Outport
  wires:
  Add1/1 -> Display2/1, Compare To Zero1/1
  Clock/1 -> Display/1, Add1/1
  Compare To Zero1/1 -> IC/1, Display5/1, Save last release time/Enable
  Constant/1 -> Add1/4  "Compensate numeric drift"
  IC/1 -> Out1/1
  Save last release time/1(n_new) -> Memory/1
  Switch/1 -> Multiply/1, Add1/3  "T_Tx"
  Multiply/1 -> Display3/1, Add1/2
  Memory/1 -> Display6/1, Multiply/2, Save last release time/1(n)
  SDTv2/1 -> Switch/2
  T_signal/1 -> Gain/1, Switch/3
  Gain/1 -> Switch/1

== system NCS_Library/Network/ETB/Subsystem2/Routing Layer/Logic 1 ==
  note: Routing
  note: Flooding
  Parameter : Inport
  Routing Table : Inport  Port=2
  FIN_Init : Inport  Port=3
  In : Inport  Port=4
  Display1 : Display
  Display4 : Display
  Entity Input Switch2 : EntityInputSwitch  InputPortMessageModes=m,m,m  OutputPortMessageModes=m  NumberInputPorts=3
      settings: InputPortMap=u1,u2,u3
  Entity Input Switch3 : EntityInputSwitch  InputPortMessageModes=m,m,m  OutputPortMessageModes=m  NumberInputPorts=3
      settings: InputPortMap=u1,u2,u3
  Entity Output Switch : EntityOutputSwitch  InputPortMessageModes=m  OutputPortMessageModes=m,m  SwitchingCriterion=From attribute  SwitchAttributeName=Route
  Entity Output Switch2 : EntityOutputSwitch  InputPortMessageModes=m  OutputPortMessageModes=m,m,m,m  NumberOutputPorts=4  SwitchingCriterion=From attribute  SwitchAttributeName=Route
      settings: OutputPortMap=o0,o1,o2,o3
  Entity Output Switch6 : EntityOutputSwitch  InputPortMessageModes=m  OutputPortMessageModes=m,m  SwitchAttributeName=Attribute1
  Entity Gate : EntityGate  InputPortMessageModes=m,m  OutputPortMessageModes=m
  Entity Replicator : EntityReplicator  InputPortMessageModes=m  OutputPortMessageModes=m,m
  Entity Replicator1 : EntityReplicator  InputPortMessageModes=m  OutputPortMessageModes=m,m
  Entity Terminator2 : EntityTerminator  InputPortMessageModes=m  NumberEntitiesArrived=on
      settings: OutputPortMap=o0
  Flooding And Reset CheckBit1 : EntityServer  InputPortMessageModes=m  OutputPortMessageModes=m  Capacity=1  ServiceTimeValue=0  EntryAction=|
      | [entity.RouterID,entity.Route,entity.MACSource] = Flooding(entity.RouterID);
      | entity.CheckBit = uint8(1);
  From own Router : EntityTerminator  InputPortMessageModes=m  NumberEntitiesArrived=on
      settings: OutputPortMap=o0
  Parameter1 : InportShadow
  Routing And Reset CheckBit : EntityServer  InputPortMessageModes=m  OutputPortMessageModes=m  Capacity=1  ServiceTimeValue=0  EntryAction=|
      | [entity.Route,entity.MACSource,entity.MACDestination,entity.RouterID] = Routing(entity.Destination,entity.RouterID);
      | entity.CheckBit = uint8(1);
  Simulink Function : $bdroot/Network/ETB/Subsystem2/Routing Layer/Logic 3/Simulink Function  SystemSampleTime=-1
  Simulink Function1 : Subsystem  TreatAsAtomicUnit=on
  Subsystem : Subsystem
  Subnet 2 : Outport
  Subnet 3 : Outport  Port=2
  wires:
  Routing And Reset CheckBit/1 -> Entity Output Switch2/1
  Entity Output Switch2/1 -> Entity Terminator2/1
  Routing Table/1 -> Simulink Function1/2(RT)
  Parameter/1 -> Simulink Function1/1(Parameter)
  Entity Output Switch6/1 -> Entity Gate/2
  Entity Terminator2/1 -> Display4/1
  FIN_Init/1 -> Subsystem/1(In1)
  Subsystem/1(Out1) -> Entity Gate/1
  Entity Gate/1 -> Routing And Reset CheckBit/1
  In/1 -> Entity Output Switch6/1
  Entity Output Switch/1 -> Entity Replicator/1
  From own Router/1 -> Display1/1
  Entity Output Switch/2 -> From own Router/1
  Entity Input Switch3/1 -> Subnet 3/1
  Entity Input Switch2/1 -> Subnet 2/1
  Entity Replicator/2 -> Entity Input Switch3/3
  Entity Replicator/1 -> Entity Input Switch2/3
  Entity Output Switch2/4 -> Entity Replicator1/1
  Entity Replicator1/2 -> Entity Input Switch3/2
  Entity Replicator1/1 -> Entity Input Switch2/2
  Entity Output Switch2/3 -> Entity Input Switch3/1
  Entity Output Switch2/2 -> Entity Input Switch2/1
  Entity Output Switch6/2 -> Flooding And Reset CheckBit1/1
  Flooding And Reset CheckBit1/1 -> Entity Output Switch/1
  Parameter1/1 -> Simulink Function/1

== system NCS_Library/Network/ETB/Subsystem2/Routing Layer/Logic 2 ==
  note: Routing
  note: Flooding
  Parameter : Inport
  Routing Table : Inport  Port=2
  FIN_Init : Inport  Port=3
  In : Inport  Port=4
  Display1 : Display
  Display4 : Display
  Entity Input Switch : EntityInputSwitch  InputPortMessageModes=m,m,m  OutputPortMessageModes=m  NumberInputPorts=3
      settings: InputPortMap=u1,u2,u3
  Entity Input Switch1 : EntityInputSwitch  InputPortMessageModes=m,m,m  OutputPortMessageModes=m  NumberInputPorts=3
      settings: InputPortMap=u1,u2,u3
  Entity Output Switch : EntityOutputSwitch  InputPortMessageModes=m  OutputPortMessageModes=m,m  SwitchingCriterion=From attribute  SwitchAttributeName=Route
  Entity Output Switch2 : EntityOutputSwitch  InputPortMessageModes=m  OutputPortMessageModes=m,m,m,m  NumberOutputPorts=4  SwitchingCriterion=From attribute  SwitchAttributeName=Route
      settings: OutputPortMap=o0,o1,o2,o3
  Entity Output Switch6 : EntityOutputSwitch  InputPortMessageModes=m  OutputPortMessageModes=m,m  SwitchAttributeName=Attribute1
  Entity Gate : EntityGate  InputPortMessageModes=m,m  OutputPortMessageModes=m
  Entity Replicator : EntityReplicator  InputPortMessageModes=m  OutputPortMessageModes=m,m
  Entity Replicator1 : EntityReplicator  InputPortMessageModes=m  OutputPortMessageModes=m,m
  Entity Terminator2 : EntityTerminator  InputPortMessageModes=m  NumberEntitiesArrived=on
      settings: OutputPortMap=o0
  Flooding And Reset CheckBit1 : EntityServer  InputPortMessageModes=m  OutputPortMessageModes=m  Capacity=1  ServiceTimeValue=0  EntryAction=|
      | [entity.RouterID,entity.Route,entity.MACSource] = Flooding(entity.RouterID);
      | entity.CheckBit = uint8(1);
  From own Router : EntityTerminator  InputPortMessageModes=m  NumberEntitiesArrived=on
      settings: OutputPortMap=o0
  Parameter1 : InportShadow
  Routing And Reset CheckBit : EntityServer  InputPortMessageModes=m  OutputPortMessageModes=m  Capacity=1  ServiceTimeValue=0  EntryAction=|
      | [entity.Route,entity.MACSource,entity.MACDestination,entity.RouterID] = Routing(entity.Destination,entity.RouterID);
      | entity.CheckBit = uint8(1);
  Simulink Function : $bdroot/Network/ETB/Subsystem2/Routing Layer/Logic 3/Simulink Function  SystemSampleTime=-1
  Simulink Function1 : Subsystem  TreatAsAtomicUnit=on
  Subsystem : Subsystem
  Subnet 1 : Outport
  Subnet 3 : Outport  Port=2
  wires:
  Routing Table/1 -> Simulink Function1/2(RT)
  Parameter/1 -> Simulink Function1/1(Parameter)
  Entity Output Switch6/1 -> Entity Gate/2
  Entity Terminator2/1 -> Display4/1
  FIN_Init/1 -> Subsystem/1(In1)
  Subsystem/1(Out1) -> Entity Gate/1
  Entity Gate/1 -> Routing And Reset CheckBit/1
  In/1 -> Entity Output Switch6/1
  Entity Output Switch6/2 -> Flooding And Reset CheckBit1/1
  Parameter1/1 -> Simulink Function/1
  Flooding And Reset CheckBit1/1 -> Entity Output Switch/1
  Entity Output Switch/1 -> Entity Replicator/1
  From own Router/1 -> Display1/1
  Entity Output Switch/2 -> From own Router/1
  Entity Input Switch1/1 -> Subnet 3/1
  Entity Input Switch/1 -> Subnet 1/1
  Entity Output Switch2/2 -> Entity Terminator2/1
  Entity Output Switch2/1 -> Entity Input Switch/1
  Entity Output Switch2/3 -> Entity Input Switch1/1
  Entity Output Switch2/4 -> Entity Replicator1/1
  Entity Replicator1/1 -> Entity Input Switch/3
  Entity Replicator1/2 -> Entity Input Switch1/2
  Entity Replicator/1 -> Entity Input Switch/2
  Entity Replicator/2 -> Entity Input Switch1/3
  Routing And Reset CheckBit/1 -> Entity Output Switch2/1

== system NCS_Library/Network/ETB/Subsystem2/Routing Layer/Logic 3 ==
  note: Routing
  note: Flooding
  Parameter : Inport
  Routing Table : Inport  Port=2
  FIN_Init : Inport  Port=3
  In : Inport  Port=4
  Display1 : Display
  Display4 : Display
  Entity Input Switch : EntityInputSwitch  InputPortMessageModes=m,m,m  OutputPortMessageModes=m  NumberInputPorts=3
      settings: InputPortMap=u1,u2,u3
  Entity Input Switch1 : EntityInputSwitch  InputPortMessageModes=m,m,m  OutputPortMessageModes=m  NumberInputPorts=3
      settings: InputPortMap=u1,u2,u3
  Entity Output Switch : EntityOutputSwitch  InputPortMessageModes=m  OutputPortMessageModes=m,m  SwitchingCriterion=From attribute  SwitchAttributeName=Route
  Entity Output Switch2 : EntityOutputSwitch  InputPortMessageModes=m  OutputPortMessageModes=m,m,m,m  NumberOutputPorts=4  SwitchingCriterion=From attribute  SwitchAttributeName=Route
      settings: OutputPortMap=o0,o1,o2,o3
  Entity Output Switch6 : EntityOutputSwitch  InputPortMessageModes=m  OutputPortMessageModes=m,m  SwitchAttributeName=Attribute1
  Entity Gate : EntityGate  InputPortMessageModes=m,m  OutputPortMessageModes=m
  Entity Replicator : EntityReplicator  InputPortMessageModes=m  OutputPortMessageModes=m,m
  Entity Replicator1 : EntityReplicator  InputPortMessageModes=m  OutputPortMessageModes=m,m
  Entity Terminator2 : EntityTerminator  InputPortMessageModes=m  NumberEntitiesArrived=on
      settings: OutputPortMap=o0
  Flooding And Reset CheckBit1 : EntityServer  InputPortMessageModes=m  OutputPortMessageModes=m  Capacity=1  ServiceTimeValue=0  EntryAction=|
      | [entity.RouterID,entity.Route,entity.MACSource] = Flooding(entity.RouterID);
      | entity.CheckBit = uint8(1);
  From own Router : EntityTerminator  InputPortMessageModes=m  NumberEntitiesArrived=on
      settings: OutputPortMap=o0
  Parameter1 : InportShadow
  Routing And Reset CheckBit : EntityServer  InputPortMessageModes=m  OutputPortMessageModes=m  Capacity=1  ServiceTimeValue=0  EntryAction=|
      | [entity.Route,entity.MACSource,entity.MACDestination,entity.RouterID] = Routing(entity.Destination,entity.RouterID);
      | entity.CheckBit = uint8(1);
  Simulink Function : Subsystem  TreatAsAtomicUnit=on
  Simulink Function1 : Subsystem  TreatAsAtomicUnit=on
  Subsystem : Subsystem
  Subnet 1 : Outport
  Subnet 2 : Outport  Port=2
  wires:
  Routing Table/1 -> Simulink Function1/2(RT)
  Parameter/1 -> Simulink Function1/1(Parameter)
  Entity Output Switch6/1 -> Entity Gate/2
  Entity Terminator2/1 -> Display4/1
  FIN_Init/1 -> Subsystem/1(In1)
  Subsystem/1(Out1) -> Entity Gate/1
  In/1 -> Entity Output Switch6/1
  Entity Output Switch6/2 -> Flooding And Reset CheckBit1/1
  Entity Input Switch/1 -> Subnet 1/1
  Entity Replicator/1 -> Entity Input Switch/2
  Entity Input Switch1/1 -> Subnet 2/1
  Entity Replicator/2 -> Entity Input Switch1/3
  Parameter1/1 -> Simulink Function/1(In1)
  Flooding And Reset CheckBit1/1 -> Entity Output Switch/1
  Entity Output Switch/1 -> Entity Replicator/1
  From own Router/1 -> Display1/1
  Entity Output Switch/2 -> From own Router/1
  Entity Gate/1 -> Routing And Reset CheckBit/1
  Entity Output Switch2/4 -> Entity Replicator1/1
  Entity Replicator1/1 -> Entity Input Switch/3
  Entity Replicator1/2 -> Entity Input Switch1/2
  Entity Output Switch2/3 -> Entity Terminator2/1
  Entity Output Switch2/1 -> Entity Input Switch/1
  Entity Output Switch2/2 -> Entity Input Switch1/1
  Routing And Reset CheckBit/1 -> Entity Output Switch2/1
